simulink model "TideVCU"  (R2021b)
settings: Solver=FixedStepDiscrete  StartTime=0.0  StopTime=10.0  RelTol=1e-3
undefined symbols (not defined in the file): dataName, enumName, enumValue, GCM, raptor_get_safe_string
libraries: Raptor_lib x93, simulink x8
(part 3 of 3)

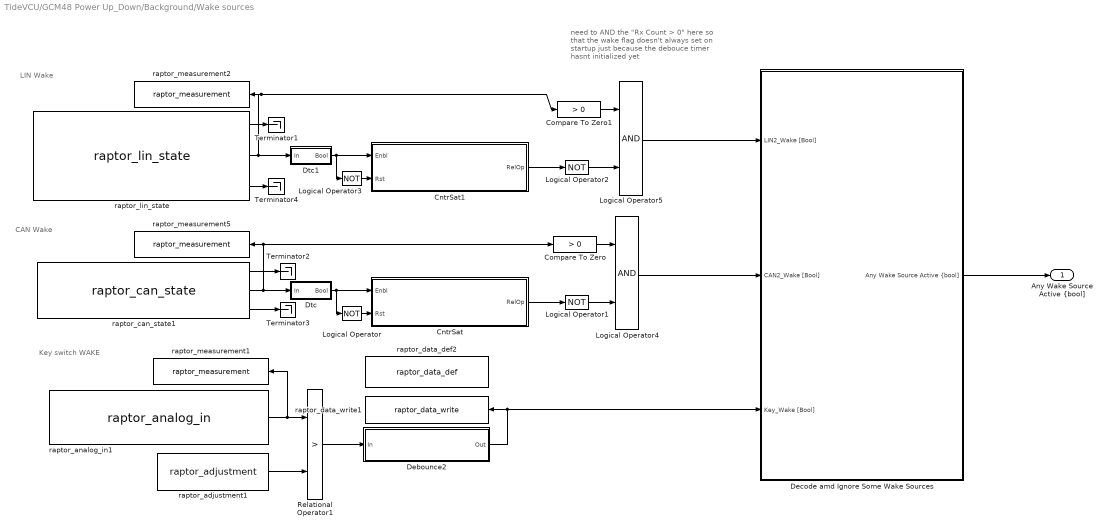
== system TideVCU/GCM48 Power Up_Down/Background/Wake sources ==
  note: CAN Wake
  note: Key switch WAKE
  note: LIN Wake
  note: need to AND the "Rx Count > 0" here so that the wake flag doesn't always set on startup just because the debouce timer hasnt initialized yet
  CntrSat : Subsystem  mask(CntrSat){init=0, inc=1, typ=uint32, relop=>=, th_nam='Wake_CAN2_SleepDelayTime', th_help='make sure this is long enough that we dont trigger a ton of EEPROM writes between messages', th_units='sec', th_gain=samptime, th_group=group}
      mask prompts: init "Initial Value (after a reset)"; inc "Increment"; typ "Data Type"; relop "Relational Operator"; th_nam "Thresh. Name"; th_help "Thresh. Help Text"; th_units "Thresh. Units"; th_gain "Thresh. Gain"; th_group "Thresh. Group"
      mask init: same as TideVCU/GCM48 Power Up_Down/Background/CntrSat2
      mask TypeOptions typ: double | single | int8 | uint8 | int16 | uint16 | int32 | uint32 | boolean
      mask TypeOptions relop: == | >= | >
      mask Display: disp(['Counter\n' typ '\n' relop ' ' th_nam]);
  CntrSat1 : Subsystem  mask(CntrSat){init=0, inc=1, typ=uint32, relop=>=, th_nam='Wake_LIN2_SleepDelayTime', th_help='make sure this is long enough that we dont trigger a ton of EEPROM writes between messages', th_units='sec', th_gain=samptime, th_group=group}
      mask prompts: init "Initial Value (after a reset)"; inc "Increment"; typ "Data Type"; relop "Relational Operator"; th_nam "Thresh. Name"; th_help "Thresh. Help Text"; th_units "Thresh. Units"; th_gain "Thresh. Gain"; th_group "Thresh. Group"
      mask init: same as TideVCU/GCM48 Power Up_Down/Background/CntrSat2
      mask TypeOptions typ: double | single | int8 | uint8 | int16 | uint16 | int32 | uint32 | boolean
      mask TypeOptions relop: == | >= | >
      mask Display: disp(['Counter\n' typ '\n' relop ' ' th_nam]);
  Compare To Zero : simulink/Logic and Bit Operations/Compare To Zero  relop=>  OutDataTypeStr=boolean
  Compare To Zero1 : simulink/Logic and Bit Operations/Compare To Zero  relop=>  OutDataTypeStr=boolean
  Debounce2 : Subsystem
  Decode amd Ignore Some Wake Sources : Subsystem
  Dtc : Subsystem  mask(Dtc){init=0, relop===}
      mask prompts: init "Initial Condition (of input):"; relop "Relational Operator"
      mask init:
      | cb = gcb;
      | 
      | % --- Parameter Setting
      | set_param([cb '/Relational Operator'], 'Operator', relop);
      mask TypeOptions relop: == | ~= | < | <= | >= | >
      mask Display: disp(['U ' relop ' U/z']);
  Dtc1 : Subsystem  mask(Dtc){init=0, relop===}
      mask prompts: init "Initial Condition (of input):"; relop "Relational Operator"
      mask init:
      | cb = gcb;
      | 
      | % --- Parameter Setting
      | set_param([cb '/Relational Operator'], 'Operator', relop);
      mask TypeOptions relop: == | ~= | < | <= | >= | >
      mask Display: disp(['U ' relop ' U/z']);
  Logical Operator{,1..3} (4 alike) : Logic  Operator=NOT  AllPortsSameDT=off  OutDataTypeStr=boolean
  Logical Operator4 : Logic  AllPortsSameDT=off  OutDataTypeStr=boolean
  Logical Operator5 : Logic  AllPortsSameDT=off  OutDataTypeStr=boolean
  Relational Operator1 : RelationalOperator  Operator=>  OutDataTypeStr=boolean  RndMeth=Simplest
  Terminator{1..4} (4 alike) : Terminator
  raptor_adjustment1 : Raptor_lib/Data Storage/raptor_adjustment  paramName='WAKE_INPUT1_Threshold'  nameSource=Parameter  initValue=1200  dataType=uint16  storage=NonVolatile (EEPROM)  calDispType=Number  calEnum={'False', 'True'}  calGain=1  calOffset=0.0  calMax=inf  calMin=-inf  calFormat='-1'  calUnit='V'  calHelp='The value of WAKE_INPUT1 analog to set key switch to true.'  calAccess=4  calFunction=group  calDispHeaders=off  calColHeaders={'Col1' 'Col2' 'Col3'}  calRowHeaders={'Row1' 'Row2' 'Row3'}
      settings: SourceProductName=Raptor
  raptor_analog_in1 : Raptor_lib/Input & Output/raptor_analog_in  resourceValues=DG1|DG2|DG3|DG4|AN1|AN2|AN3|AN4|AN5|AN6|AN7|AN8|AN9|AN10|AN11|AN12|WAKE_INPUT1|(None)  resource=WAKE_INPUT1  pullUDValues=[]  pullUD=[]  rangeValues=[]  range=[]  filterrateValues=[]  filterrate='RAPTOR MASK DEFAULT'  resolutionValues=[]  resolution=[]
      settings: SourceProductName=Raptor
  raptor_can_state1 : Raptor_lib/CAN/raptor_can_state  resourceValues=CAN1|CAN2|CAN3|CAN4|CAN5|CAN6|(None)  resource=CAN2  errOut='RAPTOR MASK DEFAULT'
      settings: SourceProductName=Raptor
  raptor_data_def2 : Raptor_lib/Data Storage/raptor_data_def  dataName='KeySw_Bgnd'  initValue=0  dataType=boolean  storage=Volatile (RAM)  calVisible=on  calType=Measurement  calDispType=Number  calEnum={'False', 'True'}  calGain=1.0  calOffset=0  calMin=-Inf  calMax=Inf  calFormat='-1'  calUnit='Bool'  calHelp='Key switch reading from background task'  calAccess=4  calFunction=group  calDispHeaders=off  calColHeaders={'Col1' 'Col2' 'Col3'}  calRowHeaders={'Row1' 'Row2' 'Row3'}
      settings: SourceProductName=Raptor
  raptor_data_write1 : Raptor_lib/Data Storage/raptor_data_write  dataName='KeySw_Bgnd'  dataShape=Scalar  idxSource=Input Port  idxRow=1  idxCol=1
      settings: SourceProductName=Raptor
  raptor_lin_state : Raptor_lib/LIN/raptor_lin_state  linBus='LIN2'
      settings: SourceProductName=Raptor
  raptor_measurement1 : Raptor_lib/Data Storage/raptor_measurement  paramName='Wake_INPUT1_Vlts'  nameSource=Parameter  calDispType=Number  calEnum={'False', 'True'}  calGain=38/4096  calOffset=0.0  calMax=inf  calMin=-inf  calFormat='-1'  calUnit=''  calHelp=''  calAccess=4  calFunction=group  calVisible=on
      settings: SourceProductName=Raptor
  raptor_measurement2 : Raptor_lib/Data Storage/raptor_measurement  paramName='Wake_LIN2_RxCount'  nameSource=Parameter  calDispType=Number  calEnum={'False', 'True'}  calGain=1.0  calOffset=0.0  calMax=inf  calMin=-inf  calFormat='-1'  calUnit=''  calHelp=''  calAccess=4  calFunction=group  calVisible=on
      settings: SourceProductName=Raptor
  raptor_measurement5 : Raptor_lib/Data Storage/raptor_measurement  paramName='Wake_CAN2_RxCount'  nameSource=Parameter  calDispType=Number  calEnum={'False', 'True'}  calGain=1.0  calOffset=0.0  calMax=inf  calMin=-inf  calFormat='-1'  calUnit=''  calHelp=''  calAccess=4  calFunction=group  calVisible=on
      settings: SourceProductName=Raptor
  "Any Wake Source Active {bool]" : Outport  VectorParamsAs1DForOutWhenUnconnected=off
  wires:
  Logical Operator5/1 -> Decode amd Ignore Some Wake Sources/1(LIN2_Wake [Bool])
  Logical Operator2/1 -> Logical Operator5/2
  Compare To Zero1/1 -> Logical Operator5/1
  Logical Operator4/1 -> Decode amd Ignore Some Wake Sources/2(CAN2_Wake [Bool])
  Compare To Zero/1 -> Logical Operator4/1
  Logical Operator1/1 -> Logical Operator4/2
  Decode amd Ignore Some Wake Sources/1("Any Wake Source Active {bool]") -> "Any Wake Source Active {bool]"/1
  raptor_can_state1/3 -> Terminator3/1
  raptor_adjustment1/1 -> Relational Operator1/2
  raptor_can_state1/1 -> Terminator2/1
  raptor_lin_state/3 -> Terminator4/1
  raptor_lin_state/1 -> Terminator1/1
  CntrSat1/1(RelOp) -> Logical Operator2/1
  Logical Operator/1 -> CntrSat/2(Rst)
  raptor_lin_state/2 -> Dtc1/1(In), raptor_measurement2/1, Compare To Zero1/1
  Logical Operator3/1 -> CntrSat1/2(Rst)
  Dtc1/1(Bool) -> Logical Operator3/1, CntrSat1/1(Enbl)
  Relational Operator1/1 -> Debounce2/1(In)
  Dtc/1(Bool) -> CntrSat/1(Enbl), Logical Operator/1
  CntrSat/1(RelOp) -> Logical Operator1/1
  raptor_analog_in1/1 -> Relational Operator1/1, raptor_measurement1/1
  Debounce2/1(Out) -> raptor_data_write1/1, Decode amd Ignore Some Wake Sources/3(Key_Wake [Bool])
  raptor_can_state1/2 -> raptor_measurement5/1, Compare To Zero/1, Dtc/1(In)

== system TideVCU/Foreground/CAN/Battery Switch/If statement for on off switch ==
  value in : Inport
  Constant2 : Constant
  Constant3 : Constant  Value=0
  If : If  IfExpression=u1 > 1200
  If Action Subsystem : Subsystem  TreatAsAtomicUnit=on
  If Action Subsystem1 : Subsystem  TreatAsAtomicUnit=on
  Merge : Merge
  Value out : Outport
  wires:
  If/2 -> If Action Subsystem1/Action
  value in/1 -> If/1
  Constant2/1 -> If Action Subsystem/1(Xa)
  If Action Subsystem1/1(Out1) -> Merge/2
  Merge/1 -> Value out/1
  If/1 -> If Action Subsystem/Action
  Constant3/1 -> If Action Subsystem1/1(Xb)
  If Action Subsystem/1(Out1) -> Merge/1

== system TideVCU/Foreground/CAN/Battery Switch/If statement for on off switch2 ==
  value in : Inport
  Constant2 : Constant
  Constant3 : Constant  Value=0
  If : If  IfExpression=u1 > 250
  If Action Subsystem : Subsystem  TreatAsAtomicUnit=on
  If Action Subsystem1 : Subsystem  TreatAsAtomicUnit=on
  Merge : Merge
  Value out : Outport
  wires:
  If/2 -> If Action Subsystem1/Action
  value in/1 -> If/1
  Constant2/1 -> If Action Subsystem/1(Xa)
  If Action Subsystem1/1(Out1) -> Merge/2
  Merge/1 -> Value out/1
  If/1 -> If Action Subsystem/Action
  Constant3/1 -> If Action Subsystem1/1(Xb)
  If Action Subsystem/1(Out1) -> Merge/1

== system TideVCU/Foreground/CAN/MCU/If statement for on off switch1 ==
  value in : Inport
  Constant2 : Constant
  Constant3 : Constant  Value=0
  If : If  IfExpression=u1 > 1200
  If Action Subsystem : Subsystem  TreatAsAtomicUnit=on
  If Action Subsystem1 : Subsystem  TreatAsAtomicUnit=on
  Merge : Merge
  Value out : Outport
  wires:
  value in/1 -> If/1
  Constant2/1 -> If Action Subsystem/1(Xa)
  If Action Subsystem1/1(Out1) -> Merge/2
  Merge/1 -> Value out/1
  If/1 -> If Action Subsystem/Action
  Constant3/1 -> If Action Subsystem1/1(Xb)
  If Action Subsystem/1(Out1) -> Merge/1
  If/2 -> If Action Subsystem1/Action

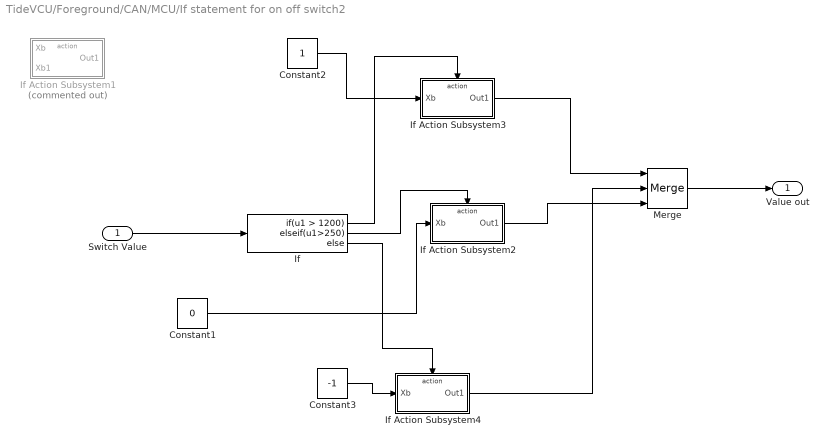
== system TideVCU/Foreground/CAN/MCU/If statement for on off switch2 ==
  Switch Value : Inport
  Constant1 : Constant  Value=0
  Constant2 : Constant
  Constant3 : Constant  Value=-1
  If : If  IfExpression=u1 > 1200  ElseIfExpressions=u1>250
  If Action Subsystem1 : Subsystem  Commented=on  TreatAsAtomicUnit=on
  If Action Subsystem2 : Subsystem  TreatAsAtomicUnit=on
  If Action Subsystem3 : Subsystem  TreatAsAtomicUnit=on
  If Action Subsystem4 : Subsystem  TreatAsAtomicUnit=on
  Merge : Merge  Inputs=3
  Value out : Outport
  wires:
  If/3 -> If Action Subsystem4/Action
  Switch Value/1 -> If/1
  If Action Subsystem4/1(Out1) -> Merge/2
  Merge/1 -> Value out/1
  Constant3/1 -> If Action Subsystem4/1(Xb)
  If/2 -> If Action Subsystem2/Action
  If Action Subsystem2/1(Out1) -> Merge/3
  Constant1/1 -> If Action Subsystem2/1(Xb)
  Constant2/1 -> If Action Subsystem3/1(Xb)
  If Action Subsystem3/1(Out1) -> Merge/1
  If/1 -> If Action Subsystem3/Action

== system TideVCU/Foreground/CAN/MCU/If statement for on off switch3 ==
  Switch Value : Inport
  Add : Sum  Inputs=+++
  Constant1 : Constant  Value=0
  Constant2 : Constant
  Constant3 : Constant  Value=-1
  If : If  IfExpression=u1 > 1200  ElseIfExpressions=u1>250
  If Action Subsystem1 : Subsystem  TreatAsAtomicUnit=on
  If Action Subsystem2 : Subsystem  TreatAsAtomicUnit=on
  If Action Subsystem3 : Subsystem  TreatAsAtomicUnit=on
  Value out : Outport
  wires:
  If/3 -> If Action Subsystem1/Action
  Switch Value/1 -> If Action Subsystem1/1(Xb), If Action Subsystem3/1(Xb), If/1
  If Action Subsystem1/1(Out1) -> Add/2
  Add/1 -> Value out/1
  Constant3/1 -> If Action Subsystem1/2(Xb1)
  If/2 -> If Action Subsystem2/Action
  If Action Subsystem2/1(Out1) -> Add/3
  Constant1/1 -> If Action Subsystem2/1(Xb)
  If/1 -> If Action Subsystem3/Action
  Constant2/1 -> If Action Subsystem3/2(Xb1)
  If Action Subsystem3/1(Out1) -> Add/1

== system TideVCU/Foreground/CAN/MCU/If statement for on off switch5 ==
  Contact value : Inport
  Add : Sum
  If : If  IfExpression=u1 < 1
  If Action Subsystem1 : Subsystem  TreatAsAtomicUnit=on
  If Action Subsystem3 : Subsystem  TreatAsAtomicUnit=on
  Value out : Outport
  wires:
  If/2 -> If Action Subsystem1/Action
  Contact value/1 -> If Action Subsystem1/1(Xb1), If Action Subsystem3/1(Xb1), If/1
  If Action Subsystem1/1(Out1) -> Add/2
  Add/1 -> Value out/1
  If/1 -> If Action Subsystem3/Action
  If Action Subsystem3/1(Out1) -> Add/1

== system TideVCU/Foreground/CAN/MCU/Left Motor ==
  Throttle : Inport
  Rudder : Inport  Port=2
  Drive Mode : Inport  Port=3
  If statement for on off switch1 : Subsystem
  Sum : Sum  Inputs=|+-
  Value out : Outport
  wires:
  Throttle/1 -> Sum/1
  Sum/1 -> If statement for on off switch1/2(Throttle)
  Rudder/1 -> Sum/2
  Drive Mode/1 -> If statement for on off switch1/1(Drive Mode swtich)
  If statement for on off switch1/1(Value out) -> Value out/1

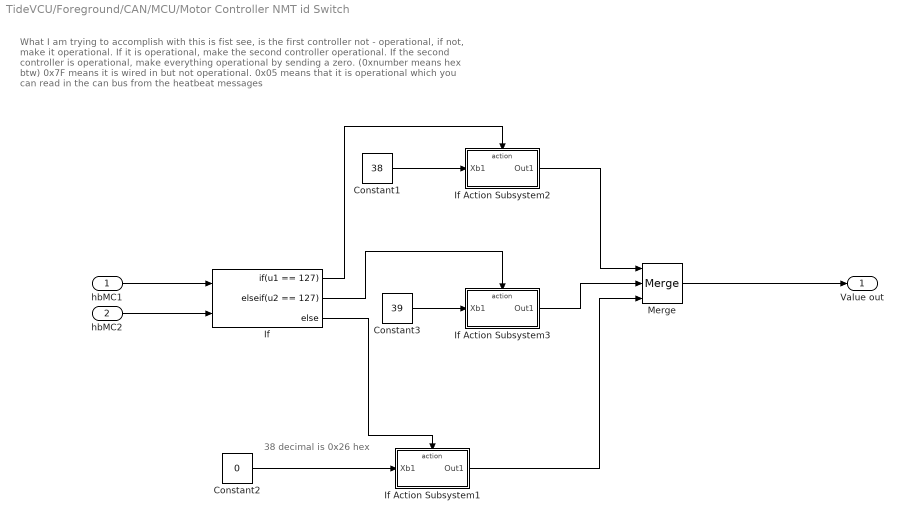
== system TideVCU/Foreground/CAN/MCU/Motor Controller NMT id Switch ==
  note: What I am trying to accomplish with this is fist see, is the first controller not - operational, if not, make it operational. If it is operational, make the second controller operational. If the second controller is operational, make everything operational by sending a zero. (0xnumber means hex btw) 0x7F means it is wired in but not operational. 0x05 means that it is operational which you can read in the can bus from the heatbeat messages
  note: 38 decimal is 0x26 hex
  hbMC1 : Inport
  hbMC2 : Inport  Port=2
  Constant1 : Constant  Value=38
  Constant2 : Constant  Value=0
  Constant3 : Constant  Value=39
  If : If  NumInputs=2  IfExpression=u1 == 127  ElseIfExpressions=u2 == 127
  If Action Subsystem1 : Subsystem  TreatAsAtomicUnit=on
  If Action Subsystem2 : Subsystem  TreatAsAtomicUnit=on
  If Action Subsystem3 : Subsystem  TreatAsAtomicUnit=on
  Merge : Merge  Inputs=3
  Value out : Outport
  wires:
  If/3 -> If Action Subsystem1/Action
  hbMC1/1 -> If/1
  If Action Subsystem1/1(Out1) -> Merge/3
  Merge/1 -> Value out/1
  If/1 -> If Action Subsystem2/Action
  If Action Subsystem2/1(Out1) -> Merge/1
  Constant1/1 -> If Action Subsystem2/1(Xb1)
  Constant2/1 -> If Action Subsystem1/1(Xb1)
  hbMC2/1 -> If/2
  If/2 -> If Action Subsystem3/Action
  Constant3/1 -> If Action Subsystem3/1(Xb1)
  If Action Subsystem3/1(Out1) -> Merge/2

== system TideVCU/Foreground/CAN/MCU/Right Motor ==
  Throttle : Inport
  Rudder : Inport  Port=2
  Drive Mode : Inport  Port=3
  Constant : Constant  Value=-1
  If statement for on off switch1 : Subsystem
  Product : Product
  Sum : Sum  Inputs=|+-
  Value out : Outport
  wires:
  Throttle/1 -> Sum/1
  Sum/1 -> If statement for on off switch1/2(Throttle)
  Rudder/1 -> Sum/2
  Drive Mode/1 -> If statement for on off switch1/1(Drive Mode swtich)
  If statement for on off switch1/1(Value out) -> Product/1
  Product/1 -> Value out/1
  Constant/1 -> Product/2

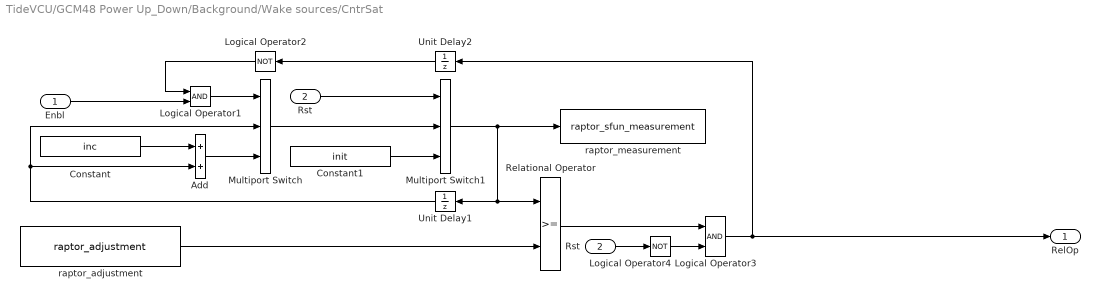
== system TideVCU/GCM48 Power Up_Down/Background/Wake sources/CntrSat ==
  Enbl : Inport
  Rst : Inport  Port=2
  Add : Sum  InputSameDT=on  OutDataTypeStr=Inherit: Same as first input
  Constant : Constant  Value=inc  OutDataTypeStr=uint32
  Constant1 : Constant  Value=init  OutDataTypeStr=uint32
  Logical Operator1 : Logic  OutDataTypeStr=boolean
  Logical Operator2 : Logic  Operator=NOT  Inputs=1  OutDataTypeStr=boolean
  Logical Operator3 : Logic  OutDataTypeStr=boolean
  Logical Operator4 : Logic  Operator=NOT  Inputs=1  OutDataTypeStr=boolean
  Multiport Switch : MultiPortSwitch  DataPortOrder=Zero-based contiguous  Inputs=2  zeroidx=on  InputSameDT=on
  Multiport Switch1 : MultiPortSwitch  DataPortOrder=Zero-based contiguous  Inputs=2  zeroidx=on  InputSameDT=on
  Relational Operator : RelationalOperator  OutDataTypeStr=boolean  RndMeth=Nearest
  "Rst " : InportShadow  Port=2
  Unit Delay1 : UnitDelay  InitialCondition=init  SampleTime=-1  HasFrameUpgradeWarning=on
  Unit Delay2 : UnitDelay  InitialCondition=boolean(0)  SampleTime=-1  HasFrameUpgradeWarning=on
  raptor_adjustment : Raptor_lib/Data Storage/raptor_adjustment  paramName=th_nam  nameSource=Parameter  initValue=5 / th_gain  dataType=uint32  storage=Calibration  calDispType=Number  calEnum={'Disabled', 'Enabled'}  calGain=th_gain  calOffset=0  calMax=inf  calMin=-inf  calFormat='0.3'  calUnit=th_units  calHelp=th_help  calAccess=4  calFunction=th_group  calDispHeaders=off  calColHeaders={'Col1' 'Col2' 'Col3'}  calRowHeaders={'Row1' 'Row2' 'Row3'}
      settings: SourceProductName=Raptor
  raptor_measurement : S-Function  FunctionName=raptor_sfun_measurement  Parameters=char({dataName,''}), uint8(calDispType), char(enumName), int32(enumValue), double(calGain), double(calOffset), double(calMax), double(calMin), char(calUnit), char(calHelp), char(calFormat), char(calFunction), char(calAccess)  SFunctionDeploymentMode=off  EnableBusSupport=off  mask(Measurement){paramName=[th_nam(1:end-3) 'Tmr'], nameSource=Parameter, calDispType=Number, calEnum={'False', 'True'}, calGain=th_gain, calOffset=0.0, calMax=inf, calMin=-inf, calFormat='0.3', calUnit=th_units, calHelp=['time that gets compared to ' th_nam], calAccess=4, calFunction=th_group, calVisible=on}
      mask prompts: paramName "Name"; nameSource "Name Source"; calDispType "Display as"; calEnum "Enumeration Definition"; calGain "Gain"; calOffset "Offset"; calMax "Max"; calMin "Min"; calFormat "Display Decimal Places"; calUnit "Unit Text"; calHelp "Help Text"; calAccess "Access Level"; calFunction "Function"; calVisible "Visible in Cal"
      mask help: This block is used to display a value in the calibration tool.
      mask init:
      | raptor_sfun_measurement_maskInit;
      settings: MoveFcn=raptor_icon_redraw(gcb);
      mask Help: eval('raptor_help(''raptor_measurement'');')
      mask TypeOptions nameSource: Parameter | Input Wire
      mask Callback nameSource: raptor_sfun_measurement_dlgCb(gcb, 'nameSource');
      mask TypeOptions calDispType: Number | Enumeration | String
      mask Callback calDispType: raptor_sfun_measurement_dlgCb(gcb, 'calDispType');
      mask TypeOptions calAccess: 4 | 3 | 2 | 1
      mask Display: raptor_sfun_measurement_icon;
  RelOp : Outport  VectorParamsAs1DForOutWhenUnconnected=off
  wires:
  Unit Delay2/1 -> Logical Operator2/1
  Rst/1 -> Multiport Switch1/1
  Logical Operator3/1 -> Unit Delay2/1, RelOp/1
  raptor_adjustment/1 -> Relational Operator/2
  Enbl/1 -> Logical Operator1/2
  Logical Operator1/1 -> Multiport Switch/1
  Add/1 -> Multiport Switch/3
  Unit Delay1/1 -> Add/2, Multiport Switch/2
  Constant/1 -> Add/1
  Multiport Switch/1 -> Multiport Switch1/2
  Constant1/1 -> Multiport Switch1/3
  Logical Operator2/1 -> Logical Operator1/1
  Multiport Switch1/1 -> raptor_measurement/1, Unit Delay1/1, Relational Operator/1
  Relational Operator/1 -> Logical Operator3/1
  Logical Operator4/1 -> Logical Operator3/2
  "Rst "/1 -> Logical Operator4/1

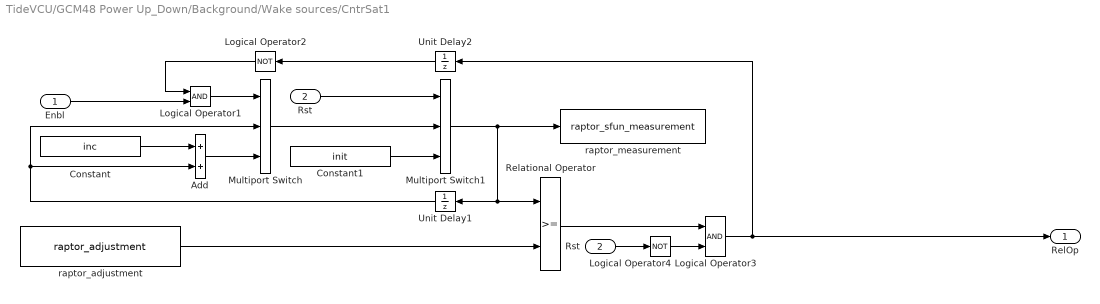
== system TideVCU/GCM48 Power Up_Down/Background/Wake sources/CntrSat1 ==
  Enbl : Inport
  Rst : Inport  Port=2
  Add : Sum  InputSameDT=on  OutDataTypeStr=Inherit: Same as first input
  Constant : Constant  Value=inc  OutDataTypeStr=uint32
  Constant1 : Constant  Value=init  OutDataTypeStr=uint32
  Logical Operator1 : Logic  OutDataTypeStr=boolean
  Logical Operator2 : Logic  Operator=NOT  Inputs=1  OutDataTypeStr=boolean
  Logical Operator3 : Logic  OutDataTypeStr=boolean
  Logical Operator4 : Logic  Operator=NOT  Inputs=1  OutDataTypeStr=boolean
  Multiport Switch : MultiPortSwitch  DataPortOrder=Zero-based contiguous  Inputs=2  zeroidx=on  InputSameDT=on
  Multiport Switch1 : MultiPortSwitch  DataPortOrder=Zero-based contiguous  Inputs=2  zeroidx=on  InputSameDT=on
  Relational Operator : RelationalOperator  OutDataTypeStr=boolean  RndMeth=Nearest
  "Rst " : InportShadow  Port=2
  Unit Delay1 : UnitDelay  InitialCondition=init  SampleTime=-1  HasFrameUpgradeWarning=on
  Unit Delay2 : UnitDelay  InitialCondition=boolean(0)  SampleTime=-1  HasFrameUpgradeWarning=on
  raptor_adjustment : Raptor_lib/Data Storage/raptor_adjustment  paramName=th_nam  nameSource=Parameter  initValue=5 / th_gain  dataType=uint32  storage=Calibration  calDispType=Number  calEnum={'Disabled', 'Enabled'}  calGain=th_gain  calOffset=0  calMax=inf  calMin=-inf  calFormat='0.3'  calUnit=th_units  calHelp=th_help  calAccess=4  calFunction=th_group  calDispHeaders=off  calColHeaders={'Col1' 'Col2' 'Col3'}  calRowHeaders={'Row1' 'Row2' 'Row3'}
      settings: SourceProductName=Raptor
  raptor_measurement : S-Function  FunctionName=raptor_sfun_measurement  Parameters=char({dataName,''}), uint8(calDispType), char(enumName), int32(enumValue), double(calGain), double(calOffset), double(calMax), double(calMin), char(calUnit), char(calHelp), char(calFormat), char(calFunction), char(calAccess)  SFunctionDeploymentMode=off  EnableBusSupport=off  mask(Measurement){paramName=[th_nam(1:end-3) 'Tmr'], nameSource=Parameter, calDispType=Number, calEnum={'False', 'True'}, calGain=th_gain, calOffset=0.0, calMax=inf, calMin=-inf, calFormat='0.3', calUnit=th_units, calHelp=['time that gets compared to ' th_nam], calAccess=4, calFunction=th_group, calVisible=on}
      mask prompts: paramName "Name"; nameSource "Name Source"; calDispType "Display as"; calEnum "Enumeration Definition"; calGain "Gain"; calOffset "Offset"; calMax "Max"; calMin "Min"; calFormat "Display Decimal Places"; calUnit "Unit Text"; calHelp "Help Text"; calAccess "Access Level"; calFunction "Function"; calVisible "Visible in Cal"
      mask help: This block is used to display a value in the calibration tool.
      mask init:
      | raptor_sfun_measurement_maskInit;
      settings: MoveFcn=raptor_icon_redraw(gcb);
      mask Help: eval('raptor_help(''raptor_measurement'');')
      mask TypeOptions nameSource: Parameter | Input Wire
      mask Callback nameSource: raptor_sfun_measurement_dlgCb(gcb, 'nameSource');
      mask TypeOptions calDispType: Number | Enumeration | String
      mask Callback calDispType: raptor_sfun_measurement_dlgCb(gcb, 'calDispType');
      mask TypeOptions calAccess: 4 | 3 | 2 | 1
      mask Display: raptor_sfun_measurement_icon;
  RelOp : Outport  VectorParamsAs1DForOutWhenUnconnected=off
  wires:
  "Rst "/1 -> Logical Operator4/1
  Logical Operator4/1 -> Logical Operator3/2
  Relational Operator/1 -> Logical Operator3/1
  Multiport Switch1/1 -> Relational Operator/1, Unit Delay1/1, raptor_measurement/1
  Logical Operator2/1 -> Logical Operator1/1
  Constant1/1 -> Multiport Switch1/3
  Multiport Switch/1 -> Multiport Switch1/2
  Constant/1 -> Add/1
  Unit Delay1/1 -> Multiport Switch/2, Add/2
  Add/1 -> Multiport Switch/3
  Logical Operator1/1 -> Multiport Switch/1
  Enbl/1 -> Logical Operator1/2
  raptor_adjustment/1 -> Relational Operator/2
  Logical Operator3/1 -> RelOp/1, Unit Delay2/1
  Rst/1 -> Multiport Switch1/1
  Unit Delay2/1 -> Logical Operator2/1

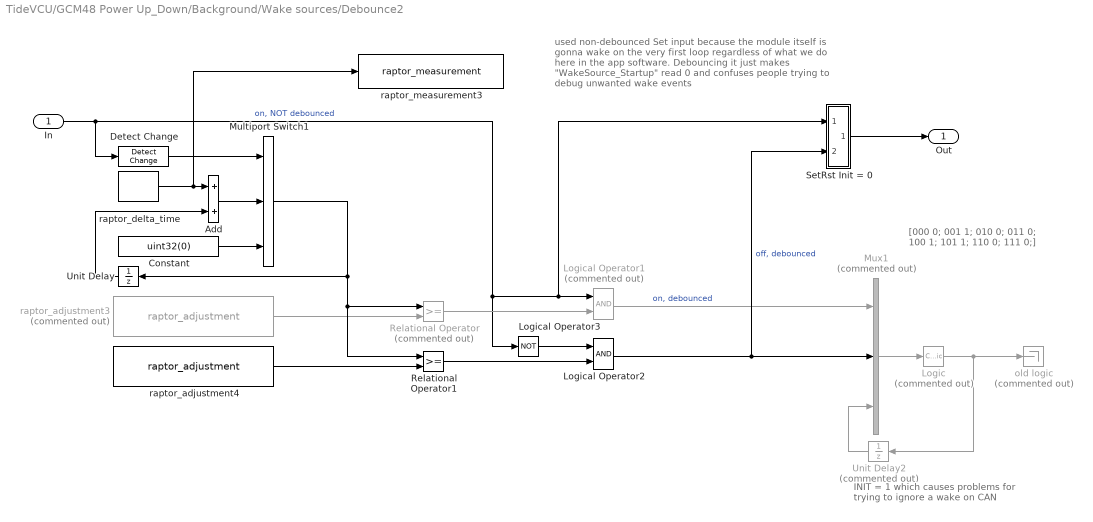
== system TideVCU/GCM48 Power Up_Down/Background/Wake sources/Debounce2 ==
  note: used non-debounced Set input because the module itself is gonna wake on the very first loop regardless of what we do here in the app software. Debouncing it just makes "WakeSource_Startup" read 0 and confuses people trying to debug unwanted wake events
  note: INIT = 1 which causes problems for trying to ignore a wake on CAN
  note: [000		0;
      |  001		1;
      |  010		0;
      |  011		0;
      |  100		1;
      |  101		1;
      |  110		0;
      |  111		0;]
  In : Inport
  Add : Sum
  Constant : Constant  Value=uint32(0)
  Detect Change : simulink/Logic and Bit Operations/Detect Change  vinit=0  OutDataTypeStr=boolean
  Logic : CombinatorialLogic  Commented=on  TruthTable=[0;1;0;0;1;1;0;0]
  Logical Operator1 : Logic  Commented=on  AllPortsSameDT=off  OutDataTypeStr=boolean
  Logical Operator2 : Logic  AllPortsSameDT=off  OutDataTypeStr=boolean
  Logical Operator3 : Logic  Operator=NOT  Inputs=1  AllPortsSameDT=off  OutDataTypeStr=boolean
  Multiport Switch1 : MultiPortSwitch  DataPortOrder=Zero-based contiguous  Inputs=2  zeroidx=on
  Mux1 : Mux  Commented=on  Inputs=3
  Relational Operator : RelationalOperator  Commented=on  OutDataTypeStr=boolean  RndMeth=Nearest
  Relational Operator1 : RelationalOperator  OutDataTypeStr=boolean  RndMeth=Nearest
  SetRst Init = 0 : Subsystem  mask(SetRst){init=0}
      mask prompts: init "Initial Condition (of output):"
      mask Display:
      | port_label('input', 1, 'S');
      | port_label('input', 2, 'R');
  Unit Delay : UnitDelay  InitialCondition=1  SampleTime=-1  HasFrameUpgradeWarning=on
  Unit Delay2 : UnitDelay  Commented=on  InitialCondition=1  SampleTime=-1  HasFrameUpgradeWarning=on
  old logic : Terminator  Commented=on
  raptor_adjustment3 : Raptor_lib/Data Storage/raptor_adjustment  Commented=on  paramName='KeySwHiTimeThr'  nameSource=Parameter  initValue=200  dataType=uint32  storage=Calibration  calDispType=Number  calEnum={'Active Low', 'Active High'}  calGain=1  calOffset=0  calMax=inf  calMin=-inf  calFormat='-1'  calUnit='milliseconds'  calHelp='State high time threshold'  calAccess=4  calFunction=group  calDispHeaders=off  calColHeaders={'Col1' 'Col2' 'Col3'}  calRowHeaders={'Row1' 'Row2' 'Row3'}
      settings: SourceProductName=Raptor
  raptor_adjustment4 : Raptor_lib/Data Storage/raptor_adjustment  paramName='KeySwLoTimeThr'  nameSource=Parameter  initValue=200  dataType=uint32  storage=Calibration  calDispType=Number  calEnum={'Active Low', 'Active High'}  calGain=1  calOffset=0  calMax=inf  calMin=-inf  calFormat='-1'  calUnit='milliseconds'  calHelp='State low time threshold'  calAccess=4  calFunction=group  calDispHeaders=off  calColHeaders={'Col1' 'Col2' 'Col3'}  calRowHeaders={'Row1' 'Row2' 'Row3'}
      settings: SourceProductName=Raptor
  raptor_delta_time : Raptor_lib/Triggers/raptor_delta_time  unit=milliseconds
      settings: SourceProductName=Raptor
  raptor_measurement3 : Raptor_lib/Data Storage/raptor_measurement  paramName='dt_read'  nameSource=Parameter  calDispType=Number  calEnum={'False', 'True'}  calGain=1.0  calOffset=0.0  calMax=inf  calMin=-inf  calFormat='-1'  calUnit=''  calHelp=''  calAccess=4  calFunction=group  calVisible=on
      settings: SourceProductName=Raptor
  Out : Outport  VectorParamsAs1DForOutWhenUnconnected=off
  wires:
  SetRst Init = 0/1(Bool) -> Out/1
  raptor_adjustment3/1 -> Relational Operator/2
  raptor_adjustment4/1 -> Relational Operator1/2
  raptor_delta_time/1 -> raptor_measurement3/1, Add/1
  Unit Delay/1 -> Add/2
  Logic/1 -> Unit Delay2/1, old logic/1
  Relational Operator1/1 -> Logical Operator2/2
  Constant/1 -> Multiport Switch1/3
  Add/1 -> Multiport Switch1/2
  Multiport Switch1/1 -> Relational Operator1/1, Relational Operator/1, Unit Delay/1
  In/1 -> Logical Operator3/1, Logical Operator1/1, SetRst Init = 0/1(Set), Detect Change/1  "on, NOT debounced"
  Unit Delay2/1 -> Mux1/3
  Mux1/1 -> Logic/1
  Logical Operator1/1 -> Mux1/1  "on, debounced"
  Logical Operator2/1 -> SetRst Init = 0/2(Rst), Mux1/2  "off, debounced"
  Relational Operator/1 -> Logical Operator1/2
  Logical Operator3/1 -> Logical Operator2/1
  Detect Change/1 -> Multiport Switch1/1

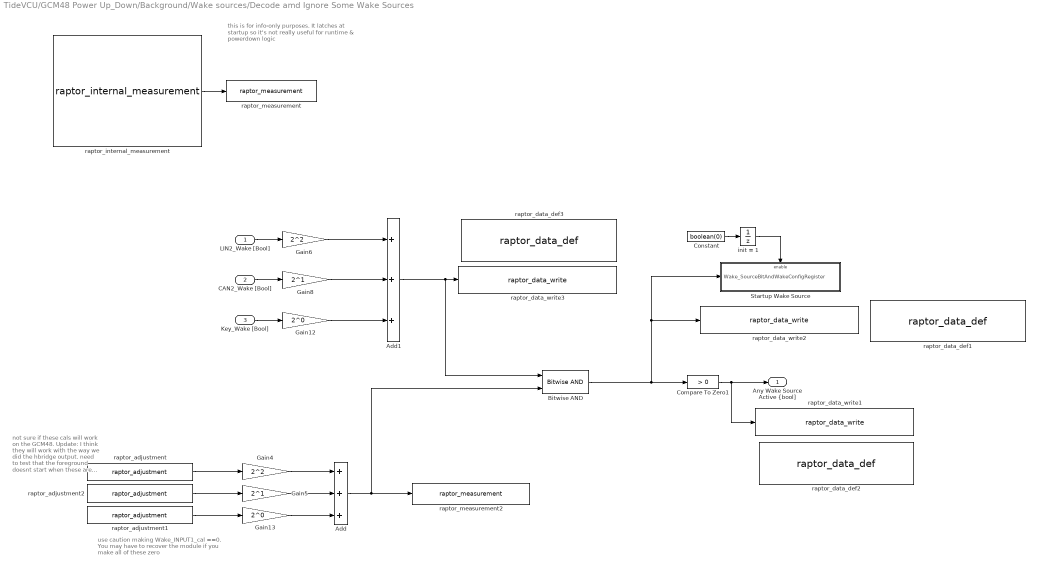
== system TideVCU/GCM48 Power Up_Down/Background/Wake sources/Decode amd Ignore Some Wake Sources ==
  note: this is for info-only purposes. It latches at startup so it's not really useful for runtime & powerdown logic
  note: not sure if these cals will work on the GCM48. Update: I think they will work with the way we did the hbridge output. need to test that the foreground doesnt start when these are zero
  note: use caution making Wake_INPUT1_cal ==0. You may have to recover the module if you make all of these zero
  LIN2_Wake [Bool] : Inport
  CAN2_Wake [Bool] : Inport  Port=2
  Key_Wake [Bool] : Inport  Port=3
  Add : Sum  Inputs=3  OutDataTypeStr=uint16
  Add1 : Sum  Inputs=3  OutDataTypeStr=uint16
  Bitwise AND : simulink/Logic and Bit Operations/Bitwise Operator  logicop=AND  UseBitMask=off  NumInputPorts=2  BitMask=bin2dec('11011001')  BitMaskRealWorld=Stored Integer
  Compare To Zero1 : simulink/Logic and Bit Operations/Compare To Zero  relop=>  OutDataTypeStr=boolean
  Constant : Constant  Value=boolean(0)
  Gain12 : Gain  Gain=2^0  OutDataTypeStr=uint16
  Gain13 : Gain  Gain=2^0  OutDataTypeStr=uint16
  Gain4 : Gain  Gain=2^2  OutDataTypeStr=uint16
  Gain5 : Gain  Gain=2^1  OutDataTypeStr=uint16
  Gain6 : Gain  Gain=2^2  OutDataTypeStr=uint16
  Gain8 : Gain  Gain=2^1  OutDataTypeStr=uint16
  Startup Wake Source : Subsystem  TreatAsAtomicUnit=on
  init = 1 : UnitDelay  InitialCondition=1  SampleTime=-1  HasFrameUpgradeWarning=on
  raptor_adjustment : Raptor_lib/Data Storage/raptor_adjustment  paramName='GCM48Wake_LIN2_cal'  nameSource=Parameter  initValue=0  dataType=boolean  storage=Calibration  calDispType=Number  calEnum={'False', 'True'}  calGain=1.0  calOffset=0.0  calMax=inf  calMin=-inf  calFormat='-1'  calUnit='bool'  calHelp='1 configures the module to wake via this input, 0 ignores this input'  calAccess=4  calFunction=group  calDispHeaders=off  calColHeaders={'Col1' 'Col2' 'Col3'}  calRowHeaders={'Row1' 'Row2' 'Row3'}
      settings: SourceProductName=Raptor
  raptor_adjustment1 : Raptor_lib/Data Storage/raptor_adjustment  paramName='GCM48Wake_INPUT1_cal'  nameSource=Parameter  initValue=1  dataType=boolean  storage=Calibration  calDispType=Number  calEnum={'False', 'True'}  calGain=1.0  calOffset=0.0  calMax=inf  calMin=-inf  calFormat='-1'  calUnit='bool'  calHelp='1 configures the module to wake via this input, 0 ignores this input'  calAccess=4  calFunction=group  calDispHeaders=off  calColHeaders={'Col1' 'Col2' 'Col3'}  calRowHeaders={'Row1' 'Row2' 'Row3'}
      settings: SourceProductName=Raptor
  raptor_adjustment2 : Raptor_lib/Data Storage/raptor_adjustment  paramName='GCM48Wake_CAN2_cal'  nameSource=Parameter  initValue=0  dataType=boolean  storage=Calibration  calDispType=Number  calEnum={'False', 'True'}  calGain=1.0  calOffset=0.0  calMax=inf  calMin=-inf  calFormat='-1'  calUnit='bool'  calHelp='1 configures the module to wake via this input, 0 ignores this input'  calAccess=4  calFunction=group  calDispHeaders=off  calColHeaders={'Col1' 'Col2' 'Col3'}  calRowHeaders={'Row1' 'Row2' 'Row3'}
      settings: SourceProductName=Raptor
  raptor_data_def1 : Raptor_lib/Data Storage/raptor_data_def  dataName='Wake_SourceBitAndWakeConfigRegister'  initValue=0  dataType=uint16  storage=Volatile (RAM)  calVisible=on  calType=Measurement  calDispType=Number  calEnum={'False', 'True'}  calGain=1.0  calOffset=0  calMin=-inf  calMax=inf  calFormat='-1'  calUnit=''  calHelp=''  calAccess=2  calFunction=group  calDispHeaders=off  calColHeaders={'Col1' 'Col2' 'Col3'}  calRowHeaders={'Row1' 'Row2' 'Row3'}
      settings: SourceProductName=Raptor
  raptor_data_def2 : Raptor_lib/Data Storage/raptor_data_def  dataName='Wake_AnyWakeSourceActive'  initValue=0  dataType=boolean  storage=Volatile (RAM)  calVisible=on  calType=Measurement  calDispType=Number  calEnum={'False', 'True'}  calGain=1.0  calOffset=0  calMin=-inf  calMax=inf  calFormat='-1'  calUnit='any wake source is keeping the module alive'  calHelp='bool'  calAccess=2  calFunction=group  calDispHeaders=off  calColHeaders={'Col1' 'Col2' 'Col3'}  calRowHeaders={'Row1' 'Row2' 'Row3'}
      settings: SourceProductName=Raptor
  raptor_data_def3 : Raptor_lib/Data Storage/raptor_data_def  dataName='WakeSource_Current'  initValue=0  dataType=uint16  storage=Volatile (RAM)  calVisible=on  calType=Measurement  calDispType=Number  calEnum={'False', 'True'}  calGain=1.0  calOffset=0  calMin=-inf  calMax=inf  calFormat='-1'  calUnit='wake source at the current instant'  calHelp=''  calAccess=2  calFunction=group  calDispHeaders=off  calColHeaders={'Col1' 'Col2' 'Col3'}  calRowHeaders={'Row1' 'Row2' 'Row3'}
      settings: SourceProductName=Raptor
  raptor_data_write1 : Raptor_lib/Data Storage/raptor_data_write  dataName='Wake_AnyWakeSourceActive'  dataShape=Scalar  idxSource=Input Port  idxRow=1  idxCol=1
      settings: SourceProductName=Raptor
  raptor_data_write2 : Raptor_lib/Data Storage/raptor_data_write  dataName='Wake_SourceBitAndWakeConfigRegister'  dataShape=Scalar  idxSource=Input Port  idxRow=1  idxCol=1
      settings: SourceProductName=Raptor
  raptor_data_write3 : Raptor_lib/Data Storage/raptor_data_write  dataName='WakeSource_Current'  dataShape=Scalar  idxSource=Input Port  idxRow=1  idxCol=1
      settings: SourceProductName=Raptor
  raptor_internal_measurement : Raptor_lib/Input & Output/raptor_internal_measurement  resourceValues=OUTPUT1_VFB|OUTPUT2_VFB|OUTPUT3_VFB|OUTPUT4_VFB|OUTPUT5_VFB|OUTPUT6_VFB|OUTPUT7_VFB|OUTPUT8_VFB|OUTPUT11_VFB|OUTPUT12_VFB|OUTPUT13_VFB|OUTPUT14_VFB|OUTPUT15_VFB|OUTPUT2_DFB|OUTPUT3_DFB|HBRIDGE9_10_DFB|OUTPUT2_IFB|OUTPUT3_IFB|HBRIDGE9_10_IFB|SENS_SUPPLY1_VFB|SENS_SUPPLY2_VFB|NTC_TEMP|WAKE_SOURCE|(None)  resource=WAKE_SOURCE  out_eng=0  soft_filter=1  out_bool=0
      settings: SourceProductName=Raptor
  raptor_measurement : Raptor_lib/Data Storage/raptor_measurement  paramName='WakeSource_RaptorIntrnlMeas'  nameSource=Parameter  calDispType=Number  calEnum={'False', 'True'}  calGain=1.0  calOffset=0.0  calMax=inf  calMin=-inf  calFormat='-1'  calUnit='wake source at startup... kinda. it often reads that LIN work the module even if the LIN bus isnt connected.'  calHelp=''  calAccess=4  calFunction=group  calVisible=on
      settings: SourceProductName=Raptor
  raptor_measurement2 : Raptor_lib/Data Storage/raptor_measurement  paramName='WakeConfigRegister'  nameSource=Parameter  calDispType=Number  calEnum={'False', 'True'}  calGain=1.0  calOffset=0.0  calMax=inf  calMin=-inf  calFormat='-1'  calUnit='register'  calHelp=''  calAccess=4  calFunction=group  calVisible=on
      settings: SourceProductName=Raptor
  "Any Wake Source Active {bool]" : Outport  VectorParamsAs1DForOutWhenUnconnected=off
  wires:
  Key_Wake [Bool]/1 -> Gain12/1
  init = 1/1 -> Startup Wake Source/Enable
  Constant/1 -> init = 1/1
  Compare To Zero1/1 -> "Any Wake Source Active {bool]"/1, raptor_data_write1/1
  LIN2_Wake [Bool]/1 -> Gain6/1
  CAN2_Wake [Bool]/1 -> Gain8/1
  raptor_adjustment1/1 -> Gain13/1
  Gain13/1 -> Add/3
  Gain12/1 -> Add1/3
  Add1/1 -> raptor_data_write3/1, Bitwise AND/1
  Gain6/1 -> Add1/1
  Gain8/1 -> Add1/2
  Bitwise AND/1 -> raptor_data_write2/1, Startup Wake Source/1(Wake_SourceBitAndWakeConfigRegister), Compare To Zero1/1
  raptor_adjustment2/1 -> Gain5/1
  Gain5/1 -> Add/2
  Add/1 -> raptor_measurement2/1, Bitwise AND/2
  raptor_internal_measurement/1 -> raptor_measurement/1
  raptor_adjustment/1 -> Gain4/1
  Gain4/1 -> Add/1

== system TideVCU/GCM48 Power Up_Down/Background/Wake sources/Dtc ==
  In : Inport
  Delay Input1 : UnitDelay  Description=Store in Global RAM  DisableCoverage=on  InitialCondition=init  SampleTime=-1  HasFrameUpgradeWarning=on
  Relational Operator : RelationalOperator  Operator===  OutDataTypeStr=boolean  RndMeth=Nearest  InputSameDT=on
  Bool : Outport  InitialOutput=0  VectorParamsAs1DForOutWhenUnconnected=off
  wires:
  In/1 -> Delay Input1/1, Relational Operator/1
  Delay Input1/1 -> Relational Operator/2
  Relational Operator/1 -> Bool/1

== system TideVCU/GCM48 Power Up_Down/Background/Wake sources/Dtc1 ==
  In : Inport
  Delay Input1 : UnitDelay  Description=Store in Global RAM  DisableCoverage=on  InitialCondition=init  SampleTime=-1  HasFrameUpgradeWarning=on
  Relational Operator : RelationalOperator  Operator===  OutDataTypeStr=boolean  RndMeth=Nearest  InputSameDT=on
  Bool : Outport  InitialOutput=0  VectorParamsAs1DForOutWhenUnconnected=off
  wires:
  Relational Operator/1 -> Bool/1
  Delay Input1/1 -> Relational Operator/2
  In/1 -> Relational Operator/1, Delay Input1/1

== system TideVCU/Foreground/CAN/Battery Switch/If statement for on off switch/If Action Subsystem ==
  Xa : Inport
  Action Port : ActionPort
  Out1 : Outport
  wires:
  Xa/1 -> Out1/1

== system TideVCU/Foreground/CAN/Battery Switch/If statement for on off switch/If Action Subsystem1 ==
  Xb : Inport
  Action Port : ActionPort
  Out1 : Outport
  wires:
  Xb/1 -> Out1/1

== system TideVCU/Foreground/CAN/Battery Switch/If statement for on off switch2/If Action Subsystem ==
  Xa : Inport
  Action Port : ActionPort
  Out1 : Outport
  wires:
  Xa/1 -> Out1/1

== system TideVCU/Foreground/CAN/Battery Switch/If statement for on off switch2/If Action Subsystem1 ==
  Xb : Inport
  Action Port : ActionPort
  Out1 : Outport
  wires:
  Xb/1 -> Out1/1

== system TideVCU/Foreground/CAN/MCU/If statement for on off switch1/If Action Subsystem ==
  Xa : Inport
  Action Port : ActionPort
  Out1 : Outport
  wires:
  Xa/1 -> Out1/1

== system TideVCU/Foreground/CAN/MCU/If statement for on off switch1/If Action Subsystem1 ==
  Xb : Inport
  Action Port : ActionPort
  Out1 : Outport
  wires:
  Xb/1 -> Out1/1

== system TideVCU/Foreground/CAN/MCU/If statement for on off switch2/If Action Subsystem1 ==
  Xb : Inport
  Xb1 : Inport  Port=2
  Action Port : ActionPort
  Product : Product
  Out1 : Outport
  wires:
  Xb/1 -> Product/2
  Xb1/1 -> Product/1
  Product/1 -> Out1/1

== system TideVCU/Foreground/CAN/MCU/If statement for on off switch2/If Action Subsystem2 ==
  Xb : Inport
  Action Port : ActionPort
  Out1 : Outport
  wires:
  Xb/1 -> Out1/1

== system TideVCU/Foreground/CAN/MCU/If statement for on off switch2/If Action Subsystem3 ==
  Xb : Inport
  Action Port : ActionPort
  Out1 : Outport
  wires:
  Xb/1 -> Out1/1

== system TideVCU/Foreground/CAN/MCU/If statement for on off switch2/If Action Subsystem4 ==
  Xb : Inport
  Action Port : ActionPort
  Out1 : Outport
  wires:
  Xb/1 -> Out1/1

== system TideVCU/Foreground/CAN/MCU/If statement for on off switch3/If Action Subsystem1 ==
  Xb : Inport
  Xb1 : Inport  Port=2
  Action Port : ActionPort
  Product : Product
  Out1 : Outport
  wires:
  Xb/1 -> Product/2
  Xb1/1 -> Product/1
  Product/1 -> Out1/1

== system TideVCU/Foreground/CAN/MCU/If statement for on off switch3/If Action Subsystem2 ==
  Xb : Inport
  Action Port : ActionPort
  Out1 : Outport
  wires:
  Xb/1 -> Out1/1

== system TideVCU/Foreground/CAN/MCU/If statement for on off switch3/If Action Subsystem3 ==
  Xb : Inport
  Xb1 : Inport  Port=2
  Action Port : ActionPort
  Product : Product
  Out1 : Outport
  wires:
  Xb/1 -> Product/2
  Xb1/1 -> Product/1
  Product/1 -> Out1/1

== system TideVCU/Foreground/CAN/MCU/If statement for on off switch5/If Action Subsystem1 ==
  Xb1 : Inport
  Action Port : ActionPort
  Out1 : Outport
  wires:
  Xb1/1 -> Out1/1

== system TideVCU/Foreground/CAN/MCU/If statement for on off switch5/If Action Subsystem3 ==
  Xb1 : Inport
  Action Port : ActionPort
  Transport Delay : TransportDelay  DelayTime=0.5
  Out1 : Outport
  wires:
  Xb1/1 -> Transport Delay/1
  Transport Delay/1 -> Out1/1

== system TideVCU/Foreground/CAN/MCU/Left Motor/If statement for on off switch1 ==
  Drive Mode swtich : Inport
  Throttle : Inport  Port=2
  Add : Sum  Inputs=+++
  Constant3 : Constant  Value=0
  If : If  IfExpression=u1 > 1400  ElseIfExpressions=u1<250
  If Action Subsystem : Subsystem  TreatAsAtomicUnit=on
  If Action Subsystem1 : Subsystem  TreatAsAtomicUnit=on
  If Action Subsystem2 : Subsystem  TreatAsAtomicUnit=on
  Value out : Outport
  wires:
  If Action Subsystem1/1(Out1) -> Add/2
  Add/1 -> Value out/1
  If/1 -> If Action Subsystem/Action
  Constant3/1 -> If Action Subsystem1/1(Xb)
  If Action Subsystem/1(Out1) -> Add/1
  If/3 -> If Action Subsystem1/Action
  Drive Mode swtich/1 -> If/1
  If/2 -> If Action Subsystem2/Action
  If Action Subsystem2/1(Out1) -> Add/3
  Throttle/1 -> If Action Subsystem2/1(Xa), If Action Subsystem/1(Xa)

== system TideVCU/Foreground/CAN/MCU/Motor Controller NMT id Switch/If Action Subsystem1 ==
  Xb1 : Inport
  Action Port : ActionPort
  Out1 : Outport
  wires:
  Xb1/1 -> Out1/1

== system TideVCU/Foreground/CAN/MCU/Motor Controller NMT id Switch/If Action Subsystem2 ==
  Xb1 : Inport
  Action Port : ActionPort
  Out1 : Outport
  wires:
  Xb1/1 -> Out1/1

== system TideVCU/Foreground/CAN/MCU/Motor Controller NMT id Switch/If Action Subsystem3 ==
  Xb1 : Inport
  Action Port : ActionPort
  Out1 : Outport
  wires:
  Xb1/1 -> Out1/1

== system TideVCU/Foreground/CAN/MCU/Right Motor/If statement for on off switch1 ==
  Drive Mode swtich : Inport
  Throttle : Inport  Port=2
  Add : Sum  Inputs=+++
  Constant3 : Constant  Value=0
  If : If  IfExpression=u1 > 1400  ElseIfExpressions=u1<250
  If Action Subsystem : Subsystem  TreatAsAtomicUnit=on
  If Action Subsystem1 : Subsystem  TreatAsAtomicUnit=on
  If Action Subsystem2 : Subsystem  TreatAsAtomicUnit=on
  Value out : Outport
  wires:
  If Action Subsystem1/1(Out1) -> Add/2
  Add/1 -> Value out/1
  If/1 -> If Action Subsystem/Action
  Constant3/1 -> If Action Subsystem1/1(Xb)
  If Action Subsystem/1(Out1) -> Add/1
  If/3 -> If Action Subsystem1/Action
  Drive Mode swtich/1 -> If/1
  If/2 -> If Action Subsystem2/Action
  If Action Subsystem2/1(Out1) -> Add/3
  Throttle/1 -> If Action Subsystem2/1(Xa), If Action Subsystem/1(Xa)

== system TideVCU/GCM48 Power Up_Down/Background/Wake sources/Debounce2/SetRst Init = 0 ==
  Set : Inport
  Rst : Inport  Port=2
  Constant : Constant  Value=boolean(0)
  Constant1 : Constant  Value=boolean(1)
  Multiport Switch : MultiPortSwitch  DataPortOrder=Zero-based contiguous  Inputs=2  zeroidx=on
  Multiport Switch1 : MultiPortSwitch  DataPortOrder=Zero-based contiguous  Inputs=2  zeroidx=on
  Unit Delay : UnitDelay  InitialCondition=init  SampleTime=-1  HasFrameUpgradeWarning=on
  Bool : Outport  VectorParamsAs1DForOutWhenUnconnected=off
  wires:
  Multiport Switch1/1 -> Multiport Switch/2
  Constant1/1 -> Multiport Switch1/3
  Constant/1 -> Multiport Switch/3
  Rst/1 -> Multiport Switch/1
  Set/1 -> Multiport Switch1/1
  Multiport Switch/1 -> Bool/1, Unit Delay/1
  Unit Delay/1 -> Multiport Switch1/2

== system TideVCU/GCM48 Power Up_Down/Background/Wake sources/Decode amd Ignore Some Wake Sources/Startup Wake Source ==
  Wake_SourceBitAndWakeConfigRegister : Inport
  Enable : EnablePort
  raptor_measurement : Raptor_lib/Data Storage/raptor_measurement  paramName='WakeSource_Startup'  nameSource=Parameter  calDispType=Number  calEnum={'False', 'True'}  calGain=1.0  calOffset=0.0  calMax=inf  calMin=-inf  calFormat='-1'  calUnit=''  calHelp=''  calAccess=4  calFunction=group  calVisible=on
      settings: SourceProductName=Raptor
  wires:
  Wake_SourceBitAndWakeConfigRegister/1 -> raptor_measurement/1

== system TideVCU/Foreground/CAN/MCU/Left Motor/If statement for on off switch1/If Action Subsystem ==
  Xa : Inport
  Action Port : ActionPort
  Out1 : Outport
  wires:
  Xa/1 -> Out1/1

== system TideVCU/Foreground/CAN/MCU/Left Motor/If statement for on off switch1/If Action Subsystem1 ==
  Xb : Inport
  Action Port : ActionPort
  Out1 : Outport
  wires:
  Xb/1 -> Out1/1

== system TideVCU/Foreground/CAN/MCU/Left Motor/If statement for on off switch1/If Action Subsystem2 ==
  Xa : Inport
  Action Port : ActionPort
  Constant : Constant  Value=-1
  Product : Product
  Out1 : Outport
  wires:
  Xa/1 -> Product/1
  Product/1 -> Out1/1
  Constant/1 -> Product/2

== system TideVCU/Foreground/CAN/MCU/Right Motor/If statement for on off switch1/If Action Subsystem ==
  Xa : Inport
  Action Port : ActionPort
  Out1 : Outport
  wires:
  Xa/1 -> Out1/1

== system TideVCU/Foreground/CAN/MCU/Right Motor/If statement for on off switch1/If Action Subsystem1 ==
  Xb : Inport
  Action Port : ActionPort
  Out1 : Outport
  wires:
  Xb/1 -> Out1/1

== system TideVCU/Foreground/CAN/MCU/Right Motor/If statement for on off switch1/If Action Subsystem2 ==
  Xa : Inport
  Action Port : ActionPort
  Constant : Constant  Value=-1
  Product : Product
  Out1 : Outport
  wires:
  Xa/1 -> Product/1
  Product/1 -> Out1/1
  Constant/1 -> Product/2
